simulink model "experiment_6"  (R2018b)
settings: Solver=VariableStepAuto  StartTime=0.0  StopTime=0.1  RelTol=1e-3
libraries: commutil2 x1, dspsigops x1, dspquant2 x1
settings Model: Creator=sangh  LastModifiedBy=sangh

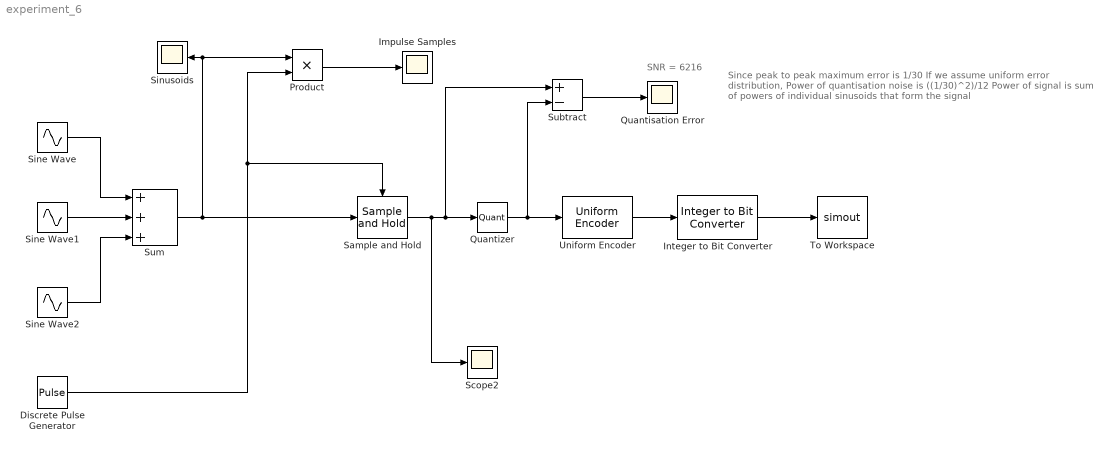
== system experiment_6 ==
  note: Since peak to peak maximum error is 1/30
      | If we assume uniform error distribution,
      | Power of quantisation noise is ((1/30)^2)/12
      | Power of signal is sum of powers of individual sinusoids that form the signal
  note: SNR = 6216
  Discrete Pulse Generator : DiscretePulseGenerator  PulseType=Time based  Period=1/8e3  PulseWidth=10
  Impulse Samples : Scope
  Integer to Bit Converter : commutil2/Integer to Bit Converter  nbits=8  signedInputValues=Signed  bitOrder=MSB first  outDtype=Inherit via internal rule
  Product : Product
  Quantisation Error : Scope
  Quantizer : Quantizer  QuantizationInterval=0.1
  Sample and Hold : dspsigops/Sample and Hold  trig=Rising edge  initCond=0  latchinput=off
  Scope2 : Scope
  Sine Wave : Sin  Frequency=2*pi*500  SampleTime=2e-6
  Sine Wave1 : Sin  Amplitude=1/3  Frequency=2*pi*1500  SampleTime=2e-6
  Sine Wave2 : Sin  Amplitude=1/5  Frequency=2*pi*2500  SampleTime=2e-6
  Sinusoids : Scope
  Subtract : Sum  Inputs=+-
  Sum : Sum  Inputs=+++
  To Workspace : ToWorkspace  VariableName=simout  SampleTime=-1
      settings: Save2DSignal=2-D array (concatenate along first dimension)
  Uniform Encoder : dspquant2/Uniform Encoder  peak=1.3  bits=8  otype=Signed integer
      settings: SourceProductName=DSP System Toolbox
  wires:
  Sine Wave1/1 -> Sum/2
  Sine Wave/1 -> Sum/1
  Sine Wave2/1 -> Sum/3
  Sum/1 -> Sample and Hold/1, Product/1, Sinusoids/1
  Discrete Pulse Generator/1 -> Sample and Hold/Trigger, Product/2
  Product/1 -> Impulse Samples/1
  Sample and Hold/1 -> Scope2/1, Subtract/1, Quantizer/1
  Quantizer/1 -> Uniform Encoder/1, Subtract/2
  Subtract/1 -> Quantisation Error/1
  Integer to Bit Converter/1 -> To Workspace/1
  Uniform Encoder/1 -> Integer to Bit Converter/1
